simulink model "sim2"  (Simulink 8.5)
settings: Solver=ode45  StartTime=0.0  StopTime=10.0  RelTol=1e-3
settings Model: Creator=alaa ahmed amer  LastModifiedBy=alaa ahmed amer
settings DataIOCC: SignalLoggingSaveFormat=Dataset
settings OptimizationCC: ExpressionDepthLimit=128
settings DebuggingCC: UnderspecifiedInitializationDetection=Simplified  MergeDetectMultiDrivingBlocksExec=error  FcnCallInpInsideContextMsg=EnableAllAsError  StateNameClashWarn=none
settings GRTTargetCC: CombineOutputUpdateFcns=on  GRTInterface=off

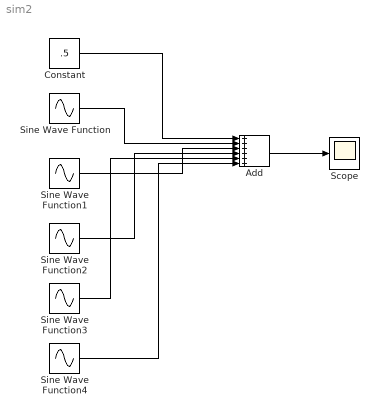
== system sim2 ==
  Add : Sum  Inputs=++++++
  Constant : Constant  Value=.5
  Scope : Scope
      settings: SampleInput=on  SampleTime=.001
  Sine Wave Function : Sin  Amplitude=2/pi  Phase=pi/2  SampleTime=0
  Sine Wave Function1 : Sin  Amplitude=-2/(pi*3)  Frequency=3  Phase=pi/2  SampleTime=0
  Sine Wave Function2 : Sin  Amplitude=2/(pi*5)  Frequency=5  Phase=pi/2  SampleTime=0
  Sine Wave Function3 : Sin  Amplitude=-2/(pi*7)  Frequency=7  Phase=pi/2  SampleTime=0
  Sine Wave Function4 : Sin  Amplitude=2/(pi*9)  Frequency=9  Phase=pi/2  SampleTime=0
  wires:
  Constant/1 -> Add/1
  Sine Wave Function/1 -> Add/2
  Sine Wave Function1/1 -> Add/3
  Sine Wave Function2/1 -> Add/4
  Sine Wave Function3/1 -> Add/5
  Sine Wave Function4/1 -> Add/6
  Add/1 -> Scope/1
